simulink model "PIDRoll"  (R2012b)
settings: Solver=ode45  StartTime=0.0  StopTime=210  RelTol=1e-3
undefined symbols (not defined in the file): DiscIntNeverNeededParam, Ts
libraries: simulink x1, slident x1
settings Model: Creator=TOSHIBA  LastModifiedBy=Carlos

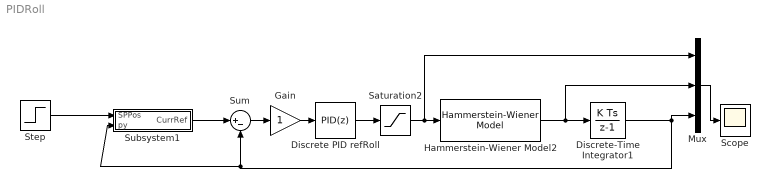
== system PIDRoll ==
  Discrete PID refRoll : simulink/Continuous/PID Controller  Controller=PID  TimeDomain=Discrete-time  SampleTime=Ts  IntegratorMethod=Forward Euler  FilterMethod=Forward Euler  Form=Parallel  P=1  I=0.002  D=0.5  N=10  InitialConditionSource=internal  InitialConditionForIntegrator=0  InitialConditionForFilter=0  ExternalReset=none  LimitOutput=off  UpperSaturationLimit=inf  LowerSaturationLimit=-inf  LinearizeAsGain=off  AntiWindupMode=none  Kb=1  TrackingMode=off  Kt=1  PParamMin=[]  PParamMax=[]  IParamMin=[]  IParamMax=[]  DParamMin=[]  DParamMax=[]  NParamMin=[]  NParamMax=[]  KbParamMin=[]  KbParamMax=[]  KtParamMin=[]  KtParamMax=[]  POutMin=[]  POutMax=[]  IOutMin=[]  IOutMax=[]  DOutMin=[]  DOutMax=[]  NOutMin=[]  NOutMax=[]  KbOutMin=[]  KbOutMax=[]  KtOutMin=[]  KtOutMax=[]  IntegratorOutMin=[]  IntegratorOutMax=[]  FilterOutMin=[]  FilterOutMax=[]  SumOutMin=[]  SumOutMax=[]  SumI1OutMin=[]  SumI1OutMax=[]  SumI2OutMin=[]  SumI2OutMax=[]  SumI3OutMin=[]  SumI3OutMax=[]  SumDOutMin=[]  SumDOutMax=[]  SaturationOutMin=[]  SaturationOutMax=[]  IntegratorContinuousStateAttributes=''  IntegratorStateMustResolveToSignalObject=off  IntegratorRTWStateStorageClass=Auto  FilterContinuousStateAttributes=''  FilterStateMustResolveToSignalObject=off  FilterRTWStateStorageClass=Auto
  Discrete-Time Integrator1 : DiscreteIntegrator  SampleTime=0.06  ICPrevOutput=DiscIntNeverNeededParam  ICPrevScaledInput=DiscIntNeverNeededParam
  Gain : Gain
  Hammerstein-Wiener Model2 : slident/Hammerstein-Wiener Model  sys=vy123_nlhw111  IC=Zero  X0i=0
  Mux : Mux  Inputs=3
  Saturation2 : Saturate  UpperLimit=1  LowerLimit=-1  SampleTime=Ts
  Scope : Scope
      settings: ShowLegends=on
  Step : Step  After=40  SampleTime=0.06
  Subsystem1 : Subsystem
  Sum : Sum  Inputs=|+-
  wires:
  Hammerstein-Wiener Model2/1 -> Mux/2, Discrete-Time Integrator1/1
  Discrete-Time Integrator1/1 -> Mux/3, Subsystem1/2(py), Sum/2
  Saturation2/1 -> Hammerstein-Wiener Model2/1, Mux/1
  Mux/1 -> Scope/1
  Discrete PID refRoll/1 -> Saturation2/1
  Sum/1 -> Gain/1
  Gain/1 -> Discrete PID refRoll/1
  Subsystem1/1(CurrRef) -> Sum/1
  Step/1 -> Subsystem1/1(SPPos)

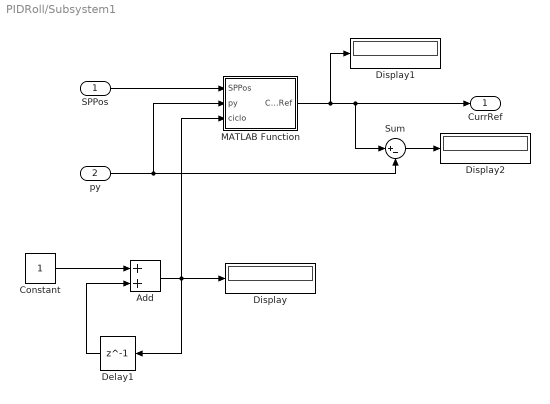
== system PIDRoll/Subsystem1 ==
  SPPos : Inport
  py : Inport  Port=2
  Add : Sum
  Constant : Constant
  Delay1 : Delay  DelayLength=1  InitialCondition=0  SampleTime=Ts
  Display : Display
  Display1 : Display
  Display2 : Display
  MATLAB Function : MATLAB Function  TreatAsAtomicUnit=on
  Sum : Sum  Inputs=|+-
  CurrRef : Outport
  wires:
  MATLAB Function/1(CurrRef) -> Display1/1, Sum/1, CurrRef/1
  SPPos/1 -> MATLAB Function/1(SPPos)
  py/1 -> Sum/2, MATLAB Function/2(py)
  Add/1 -> MATLAB Function/3(ciclo), Display/1, Delay1/1
  Delay1/1 -> Add/2
  Constant/1 -> Add/1
  Sum/1 -> Display2/1

== matlab function PIDRoll/Subsystem1/MATLAB Function ==
  data: SPPos input; py input; ciclo input; CurrRef output
function CurrRef = CalcRef(SPPos,py,ciclo)
if (SPPos>py)
    Ax=ciclo*0.0004;
else
    Ax=0;
end

CurrRef = py+Ax;
end
